simulink model "Sim_quadrotor"  (R2024a)
settings: Solver=ode4  StartTime=0.0  StopTime=18  FixedStep=sample_time_continous  RelTol=1e-3
values from neighbouring files (symbols this model uses):
  A_continuous = [0,0,0,1,0,0,0,0,0,0,0,0;      0,0,0,0,1,0,0,0,0,0,0,0;      0,0,0,0,0,1,0,0,0,0,0,0;      0,0,0,0,0,0,g * sin(alpha),g * cos(alpha),0,0,0,0;      0,0,0,0,0,0,-g * cos(alpha),g * sin(alpha),0,0,0,0;      0,0,0,0,0,0,0,0,0,0,0,0;      0,0,0,0,0,0,0,0,0,1,0,0;      0,0,0,0,0,0,0,0,0,0,1,0;      0,0,0,0,0,0,0,0,0,0,0,1;      0,0,0,0,0,0,0,0,0,0,0,0;      0,0,0,0,0,0,0,0,0,0,0,0;      0,0,0,0,0,0,0,0, ...(+8 chars)    [Main_quadrotor.m]
  A_continuous_outer = [zeros(3, 3), eye(3)     , zeros(3, 3);                       zeros(3, 3), zeros(3, 3), G          ;                       zeros(3, 3), zeros(3, 3), zeros(3, 3)]    [Main_quadrotor.m]
  B_continuous = [0,0,0,0;      0,0,0,0;      0,0,0,0;      0,0,0,0;      0,0,0,0;      1/m,1/m,1/m,1/m;      0,0,0,0;      0,0,0,0;      0,0,0,0;      inertia_true_inverse*[layout_true(2,:);-layout_true(1,:);layout_true(3,:)]]    [Main_quadrotor.m]
  B_continuous_outer = [zeros(5, 1), zeros(5, 3);                       1/m        , zeros(1, 3);                       zeros(3, 1), eye(3)     ]    [Main_quadrotor.m]
  C_inner_and_outer = eye(12)    [Main_quadrotor.m]
  DSM_val_lower_threshold_pathFG = 0    [Main_quadrotor.m]
  DSM_val_upper_threshold_pathFG = 0.01    [Main_quadrotor.m]
  goal = [2.5; 2.5; 1]    [Main_quadrotor.m]
  inner_controller_inclusion = 0    [Main_quadrotor.m]
  iter_max_pathFG = 50    [Main_quadrotor.m]
  K_lqr_outer_loop = K_lqr_outer_loop_discrete_time    [Main_quadrotor.m]
  kappa_o = 5    [Main_quadrotor.m]
  kappa_pathFG = 0.5    [Main_quadrotor.m]
  kappa_s = 2    [Main_quadrotor.m]
  MPC_max_iters = 200    [Main_quadrotor.m]
  nrotor_initial_condition = [start; zeros(9, 1)]    [Main_quadrotor.m]
  obstacle_sizes = obstacle_sizes'    [Main_quadrotor.m]
  obstacles = obstacles'    [Main_quadrotor.m]
  PathFG_max_N = 30    [Main_quadrotor.m]
  prediction_horizon_MPC = prediction_horizons_MPC(1)    [Main_quadrotor.m]
  safety_margin_universal = 0.05    [Main_quadrotor.m]
  sample_time_controller_outer = 1/10    (= 0.1)    [Main_quadrotor.m]    (also in Main_unicycle.m)
  sample_time_pathFG = sample_time_controller_outer    (= 0.1)    [Main_quadrotor.m]    (also in Main_unicycle.m)
  solver = 2    [Main_quadrotor.m]
  start = [0.1; 0.1; 0.3]    [Main_quadrotor.m]
  u_max = [thrust_max - mass_true * g; 0.5*pi; 0.5*pi; 0.5*pi]    [Main_quadrotor.m]
  u_min = [thrust_min - mass_true * g + thrust_space_saved_for_PID_inner_controller; -0.5*pi; -0.5*pi; -0.5*pi]    [Main_quadrotor.m]
undefined symbols (not defined in the file or in its folder): agent_params, agent_size, cmd_2_newtons_conversion_linear_coefficient, cmd_2_newtons_conversion_quadratic_coefficient, cmd_max, cmd_min, constr_mat, decision_variables_init, DiscIntNeverNeededParam, g, inertia_true, inertia_true_inverse, K_lqr_outer_loop_discrete_time, layout_true, mass_for_controller, mass_true, measurement_noise_accelerometer_covariance_decomposition, measurement_noise_accelerometer_mean, measurement_noise_accelerometer_seed, measurement_noise_accelerometer_var, measurement_noise_body_accelerations_inclusion_multiplier, measurement_noise_body_rates_inclusion_multiplier, measurement_noise_full_state_inclusion_multiplier, measurement_noise_full_state_mean, measurement_noise_full_state_seed, measurement_noise_full_state_var, measurement_noise_gyroscope_covariance_decomposition, measurement_noise_gyroscope_mean, measurement_noise_gyroscope_seed, measurement_noise_gyroscope_var, nrotor_vehicle_thrust_max, obs_params, P_matrix, path, pid_x_body_rate_integrator_limit, pid_x_body_rate_kp, pid_y_body_rate_integrator_limit, pid_y_body_rate_kp, pid_z_body_rate_kp, rect_obs, sample_time_controller_inner, sample_time_measurements_body_accelerations, sample_time_measurements_body_rates, sample_time_measurements_full_state, size_of_path, ssmodel, weights
libraries: simulink x15
settings Model: Creator=NewCrest Consulting  LastModifiedBy=serena
settings RTWCC: GPUComputeCapability=3.5

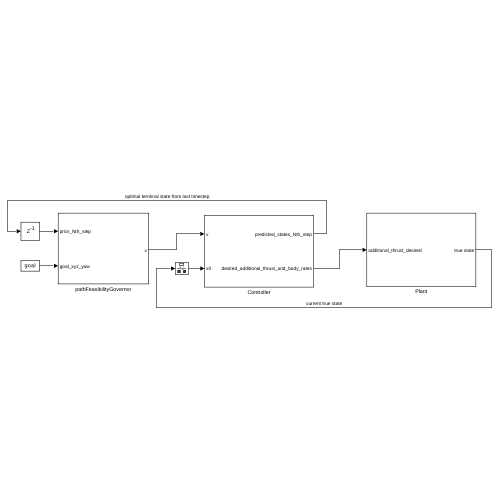
[thumbnail: Simulink's stored preview of the top-level diagram]
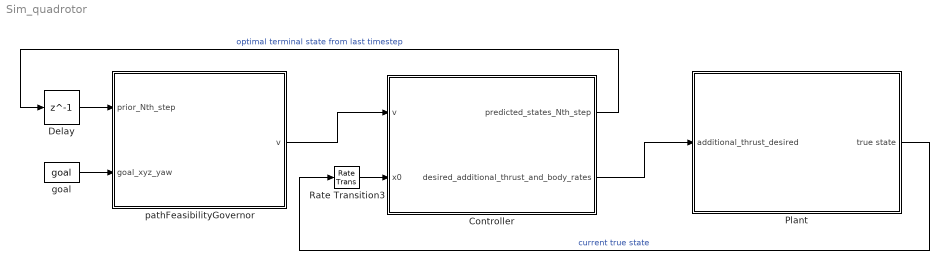
== system Sim_quadrotor ==
  Controller : Subsystem
  Delay : Delay  DelayLength=1  InitialCondition=[start;0;0;0;0;0;0]
  Plant : Subsystem
  Rate Transition3 : RateTransition  InitialCondition=[start;0;0;0;0;0;0]  OutPortSampleTime=sample_time_controller_outer
  goal : Constant  Value=goal
  pathFeasibilityGovernor : Subsystem  VariantControl=ref_source == 3
  wires:
  goal/1 -> pathFeasibilityGovernor/2(goal_xyz_yaw)
  Rate Transition3/1 -> Controller/2(x0)
  Plant/1(true state) -> Rate Transition3/1  "current true state"
  Delay/1 -> pathFeasibilityGovernor/1(prior_Nth_step)
  pathFeasibilityGovernor/1(v) -> Controller/1(v)
  Controller/1(predicted_states_Nth_step) -> Delay/1  "optimal terminal state from last timestep"
  Controller/2(desired_additional_thrust_and_body_rates) -> Plant/1(additional_thrust_desired)

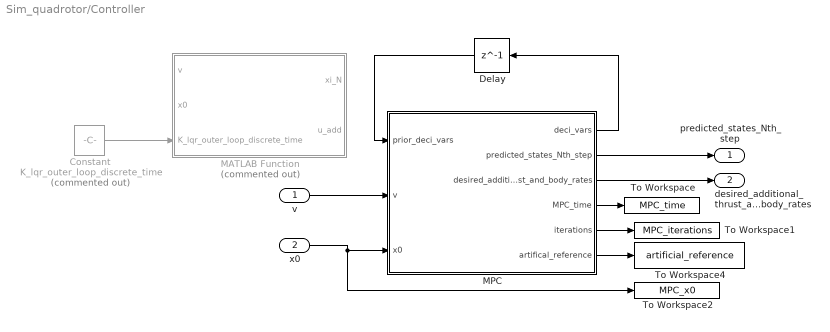
== system Sim_quadrotor/Controller ==
  v : Inport
  x0 : Inport  Port=2
  Constant : Constant  Commented=on  Value=K_lqr_outer_loop_discrete_time
  Delay : Delay  DelayLength=1  InitialCondition=decision_variables_init
  MATLAB Function : MATLAB Function  Commented=on  TreatAsAtomicUnit=on
  MPC : MATLAB Function  TreatAsAtomicUnit=on  SystemSampleTime=sample_time_controller_outer
  To Workspace : ToWorkspace  VariableName=MPC_time  SaveFormat=Timeseries  SampleTime=-1
  To Workspace1 : ToWorkspace  VariableName=MPC_iterations  SaveFormat=Timeseries  SampleTime=-1
  To Workspace2 : ToWorkspace  VariableName=MPC_x0  SaveFormat=Timeseries  SampleTime=-1
  To Workspace4 : ToWorkspace  VariableName=artificial_reference  SaveFormat=Timeseries  SampleTime=-1
  predicted_states_Nth_step : Outport
  desired_additional_thrust_and_body_rates : Outport  Port=2
  wires:
  Delay/1 -> MPC/1(prior_deci_vars)
  MPC/1(deci_vars) -> Delay/1
  v/1 -> MPC/2(v)
  MPC/2(predicted_states_Nth_step) -> predicted_states_Nth_step/1
  x0/1 -> To Workspace2/1, MPC/3(x0)
  MPC/3(desired_additional_thrust_and_body_rates) -> desired_additional_thrust_and_body_rates/1
  Constant/1 -> MATLAB Function/3(K_lqr_outer_loop_discrete_time)
  MPC/4(MPC_time) -> To Workspace/1
  MPC/5(iterations) -> To Workspace1/1
  MPC/6(artifical_reference) -> To Workspace4/1

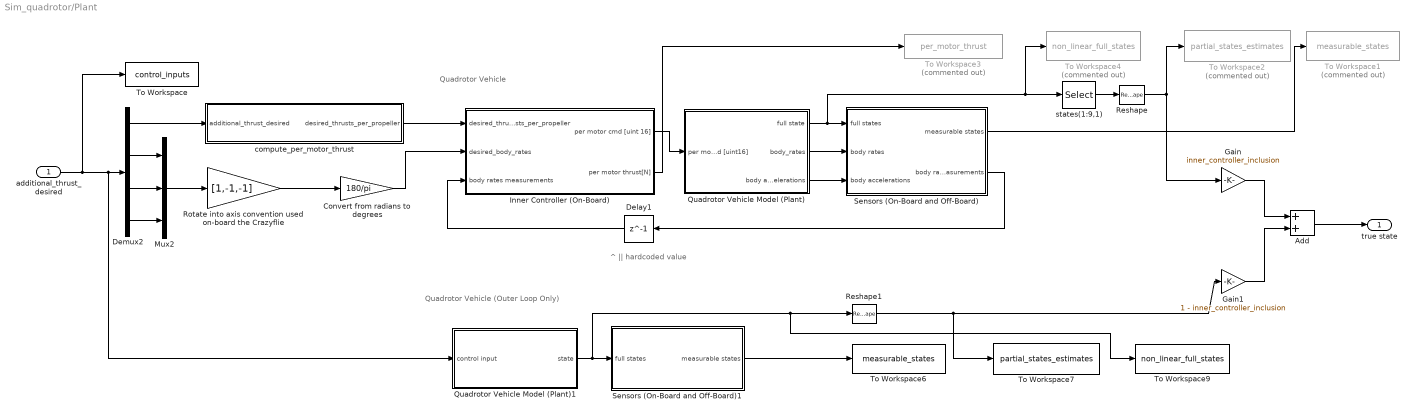
== system Sim_quadrotor/Plant ==
  note: Quadrotor Vehicle
  note: ^
      |             ||
      | hardcoded value
  note: Quadrotor Vehicle (Outer Loop Only)
  additional_thrust_desired : Inport
  Add : Sum
  Convert from radians to degrees : Gain  Gain=180/pi
  Delay1 : Delay  DelayLength=1  InitialCondition=[0;0;0]
  Demux2 : Demux
  Gain : Gain  Gain=inner_controller_inclusion
  Gain1 : Gain  Gain=1 - inner_controller_inclusion
  Inner Controller (On-Board) : Subsystem
  Mux2 : Mux  Inputs=3
  Quadrotor Vehicle Model (Plant) : Subsystem
  Quadrotor Vehicle Model (Plant)1 : Subsystem
  Reshape : Reshape  OutputDimensionality=Column vector (2-D)
  Reshape1 : Reshape  OutputDimensionality=Column vector (2-D)
  Rotate into axis convention used on-board the Crazyflie : Gain  Gain=[1,-1,-1]
  Sensors (On-Board and Off-Board) : Subsystem
  Sensors (On-Board and Off-Board)1 : Subsystem
  To Workspace : ToWorkspace  VariableName=control_inputs  SaveFormat=Timeseries  SampleTime=-1
  To Workspace1 : ToWorkspace  Commented=on  VariableName=measurable_states  SaveFormat=Timeseries  SampleTime=-1
  To Workspace2 : ToWorkspace  Commented=on  VariableName=partial_states_estimates  SaveFormat=Timeseries  SampleTime=-1
  To Workspace3 : ToWorkspace  Commented=on  VariableName=per_motor_thrust  SaveFormat=Timeseries  SampleTime=-1
  To Workspace4 : ToWorkspace  Commented=on  VariableName=non_linear_full_states  SaveFormat=Timeseries  SampleTime=-1
  To Workspace6 : ToWorkspace  VariableName=measurable_states  SaveFormat=Timeseries  SampleTime=-1
  To Workspace7 : ToWorkspace  VariableName=partial_states_estimates  SaveFormat=Timeseries  SampleTime=-1
  To Workspace9 : ToWorkspace  VariableName=non_linear_full_states  SaveFormat=Timeseries  SampleTime=-1
  compute_per_motor_thrust : MATLAB Function  TreatAsAtomicUnit=on
  states(1:9,1) : Selector  InputPortWidth=12  IndexOptions=Index vector (dialog)  Indices=[1,2,3,4,5,6,7,8,9]  OutputSizes=1
  true state : Outport
  wires:
  Sensors (On-Board and Off-Board)/1(measurable states) -> To Workspace1/1
  Quadrotor Vehicle Model (Plant)/3(body accelerations) -> Sensors (On-Board and Off-Board)/3(body accelerations)
  Inner Controller (On-Board)/2(per motor thrust[N]) -> To Workspace3/1
  Quadrotor Vehicle Model (Plant)/2(body_rates) -> Sensors (On-Board and Off-Board)/2(body rates)
  Inner Controller (On-Board)/1(per motor cmd [uint 16]) -> Quadrotor Vehicle Model (Plant)/1(per motor cmd [uint16])
  compute_per_motor_thrust/1(desired_thrusts_per_propeller) -> Inner Controller (On-Board)/1(desired_thrusts_per_propeller)
  Convert from radians to degrees/1 -> Inner Controller (On-Board)/2(desired_body_rates)
  Rotate into axis convention used on-board the Crazyflie/1 -> Convert from radians to degrees/1
  additional_thrust_desired/1 -> Quadrotor Vehicle Model (Plant)1/1(control input), Demux2/1, To Workspace/1
  Demux2/1 -> compute_per_motor_thrust/1(additional_thrust_desired)
  Demux2/2 -> Mux2/1
  Demux2/4 -> Mux2/3
  Demux2/3 -> Mux2/2
  Mux2/1 -> Rotate into axis convention used on-board the Crazyflie/1
  Quadrotor Vehicle Model (Plant)/1(full state) -> Sensors (On-Board and Off-Board)/1(full states), To Workspace4/1, states(1:9,1)/1
  Reshape/1 -> Gain/1, To Workspace2/1
  states(1:9,1)/1 -> Reshape/1
  Sensors (On-Board and Off-Board)/2(body rates measurements) -> Delay1/1
  Delay1/1 -> Inner Controller (On-Board)/3(body rates measurements)
  Sensors (On-Board and Off-Board)1/1(measurable states) -> To Workspace6/1
  Reshape1/1 -> Gain1/1, To Workspace7/1
  Quadrotor Vehicle Model (Plant)1/1(state) -> Sensors (On-Board and Off-Board)1/1(full states), Reshape1/1, To Workspace9/1
  Gain/1 -> Add/1
  Gain1/1 -> Add/2
  Add/1 -> true state/1

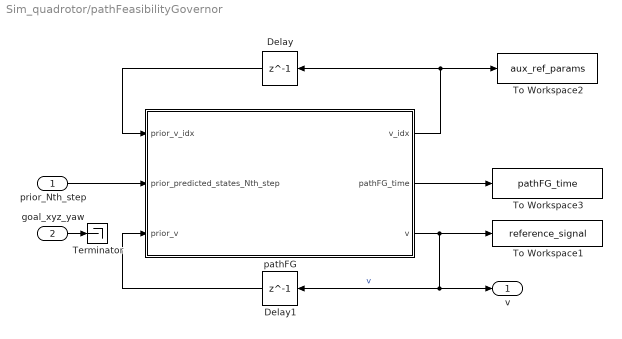
== system Sim_quadrotor/pathFeasibilityGovernor ==
  prior_Nth_step : Inport
  goal_xyz_yaw : Inport  Port=2
  Delay : Delay  DelayLength=1  InitialCondition=1
  Delay1 : Delay  DelayLength=1  InitialCondition=[start;0]
  Terminator : Terminator
  To Workspace1 : ToWorkspace  VariableName=reference_signal  SaveFormat=Timeseries  SampleTime=-1
  To Workspace2 : ToWorkspace  VariableName=aux_ref_params  SaveFormat=Timeseries  SampleTime=-1
  To Workspace3 : ToWorkspace  VariableName=pathFG_time  SaveFormat=Timeseries  SampleTime=-1
  pathFG : MATLAB Function  TreatAsAtomicUnit=on  SystemSampleTime=sample_time_pathFG
  v : Outport
  wires:
  goal_xyz_yaw/1 -> Terminator/1
  pathFG/3(v) -> To Workspace1/1, v/1, Delay1/1  "v"
  prior_Nth_step/1 -> pathFG/2(prior_predicted_states_Nth_step)
  pathFG/1(v_idx) -> Delay/1, To Workspace2/1
  Delay/1 -> pathFG/1(prior_v_idx)
  Delay1/1 -> pathFG/3(prior_v)
  pathFG/2(pathFG_time) -> To Workspace3/1

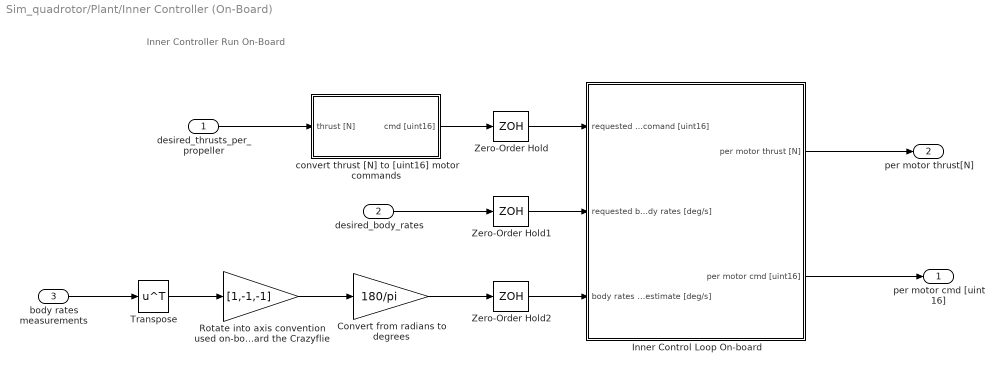
== system Sim_quadrotor/Plant/Inner Controller (On-Board) ==
  note: Inner Controller Run On-Board
  desired_thrusts_per_propeller : Inport
  desired_body_rates : Inport  Port=2
  body rates measurements : Inport  Port=3
  Convert from radians to degrees : Gain  Gain=180/pi
  Inner Control Loop On-board : Subsystem
  Rotate into axis convention used on-board the Crazyflie : Gain  Gain=[1,-1,-1]
  Transpose : Math  Operator=transpose
  Zero-Order Hold : ZeroOrderHold  SampleTime=sample_time_controller_inner
  Zero-Order Hold1 : ZeroOrderHold  SampleTime=sample_time_controller_inner
  Zero-Order Hold2 : ZeroOrderHold  SampleTime=sample_time_controller_inner
  convert thrust [N] to [uint16] motor commands : Subsystem
  per motor cmd [uint 16] : Outport
  per motor thrust[N] : Outport  Port=2
  wires:
  Inner Control Loop On-board/2(per motor cmd [uint16]) -> per motor cmd [uint 16]/1
  desired_body_rates/1 -> Zero-Order Hold1/1
  Zero-Order Hold/1 -> Inner Control Loop On-board/1(requested per motor comand [uint16])
  desired_thrusts_per_propeller/1 -> convert thrust [N] to [uint16] motor commands/1(thrust [N])
  Zero-Order Hold2/1 -> Inner Control Loop On-board/3(body rates estimate [deg/s])
  Zero-Order Hold1/1 -> Inner Control Loop On-board/2(requested body rates [deg/s])
  Inner Control Loop On-board/1(per motor thrust [N]) -> per motor thrust[N]/1
  Rotate into axis convention used on-board the Crazyflie/1 -> Convert from radians to degrees/1
  Convert from radians to degrees/1 -> Zero-Order Hold2/1
  body rates measurements/1 -> Transpose/1
  convert thrust [N] to [uint16] motor commands/1(cmd [uint16]) -> Zero-Order Hold/1
  Transpose/1 -> Rotate into axis convention used on-board the Crazyflie/1

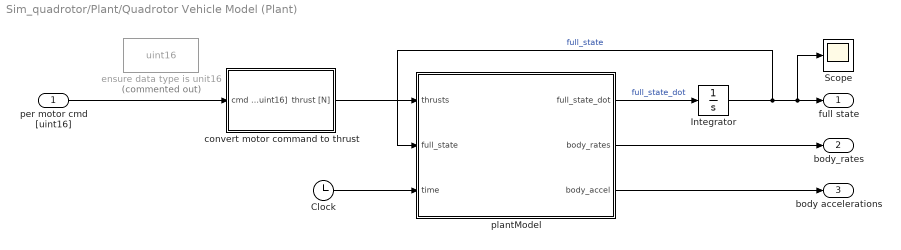
== system Sim_quadrotor/Plant/Quadrotor Vehicle Model (Plant) ==
  per motor cmd [uint16] : Inport
  Clock : Clock
  Integrator : Integrator  InitialCondition=nrotor_initial_condition
  Scope : Scope
  convert motor command to thrust : Subsystem
  ensure data type is unit16 : DataTypeConversion  Commented=on  OutDataTypeStr=uint16  SaturateOnIntegerOverflow=off  RndMeth=Floor
  plantModel : MATLAB Function  TreatAsAtomicUnit=on
  full state : Outport  VectorParamsAs1DForOutWhenUnconnected=off
  body_rates : Outport  Port=2  VectorParamsAs1DForOutWhenUnconnected=off
  body accelerations : Outport  Port=3  VectorParamsAs1DForOutWhenUnconnected=off
  wires:
  plantModel/3(body_accel) -> body accelerations/1
  convert motor command to thrust/1(thrust [N]) -> plantModel/1(thrusts)
  plantModel/2(body_rates) -> body_rates/1
  plantModel/1(full_state_dot) -> Integrator/1  "full_state_dot"
  per motor cmd [uint16]/1 -> convert motor command to thrust/1(cmd [uint16])
  Integrator/1 -> Scope/1, full state/1, plantModel/2(full_state)  "full_state"
  Clock/1 -> plantModel/3(time)

== system Sim_quadrotor/Plant/Quadrotor Vehicle Model (Plant)1 ==
  control input : Inport
  Integrator : Integrator  InitialCondition=nrotor_initial_condition(1:9)
  MATLAB Function : MATLAB Function  TreatAsAtomicUnit=on
  Scope : Scope
  state : Outport  VectorParamsAs1DForOutWhenUnconnected=off
  wires:
  control input/1 -> MATLAB Function/2(control_input)
  MATLAB Function/1(state_dot) -> Integrator/1  "state_dot"
  Integrator/1 -> Scope/1, MATLAB Function/1(state), state/1  "state"

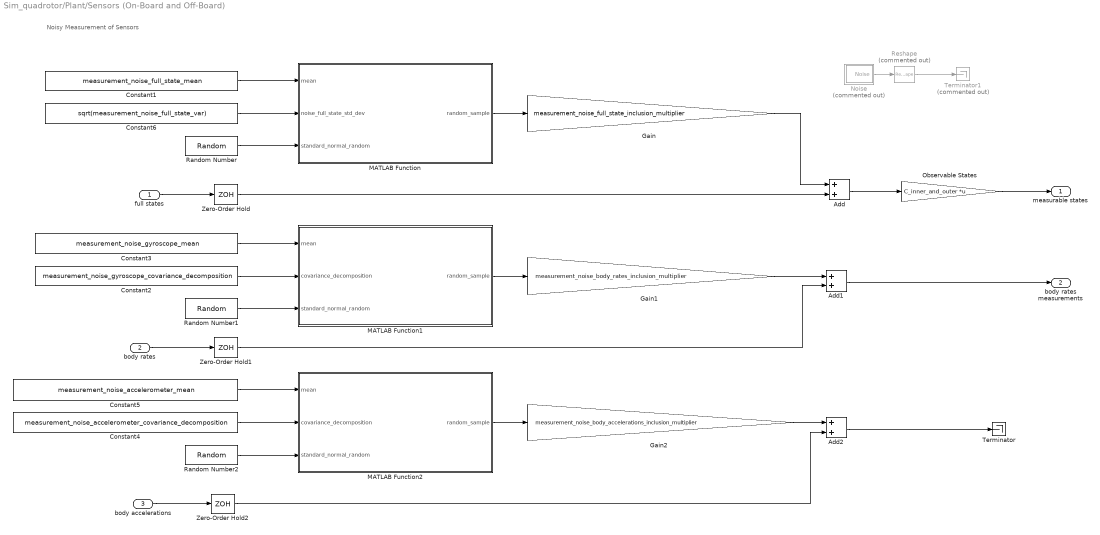
== system Sim_quadrotor/Plant/Sensors (On-Board and Off-Board) ==
  note: Noisy Measurement of Sensors
  full states : Inport
  body rates : Inport  Port=2
  body accelerations : Inport  Port=3
  Add : Sum
  Add1 : Sum
  Add2 : Sum
  Constant1 : Constant  Value=measurement_noise_full_state_mean  VectorParams1D=off
  Constant2 : Constant  Value=measurement_noise_gyroscope_covariance_decomposition
  Constant3 : Constant  Value=measurement_noise_gyroscope_mean
  Constant4 : Constant  Value=measurement_noise_accelerometer_covariance_decomposition
  Constant5 : Constant  Value=measurement_noise_accelerometer_mean
  Constant6 : Constant  Value=sqrt(measurement_noise_full_state_var)
  Gain : Gain  Gain=measurement_noise_full_state_inclusion_multiplier
  Gain1 : Gain  Gain=measurement_noise_body_rates_inclusion_multiplier
  Gain2 : Gain  Gain=measurement_noise_body_accelerations_inclusion_multiplier
  MATLAB Function : MATLAB Function  TreatAsAtomicUnit=on
  MATLAB Function1 : MATLAB Function  TreatAsAtomicUnit=on
  MATLAB Function2 : MATLAB Function  TreatAsAtomicUnit=on
  Noise : Subsystem  Commented=on
  Observable States : Gain  Gain=C_inner_and_outer  Multiplication=Matrix(K*u)
  Random Number : RandomNumber  Mean=zeros(12,1)  Variance=ones(12,1)  Seed=measurement_noise_full_state_seed  SampleTime=sample_time_measurements_full_state  VectorParams1D=off
  Random Number1 : RandomNumber  Mean=measurement_noise_gyroscope_mean  Variance=measurement_noise_gyroscope_var  Seed=measurement_noise_gyroscope_seed  SampleTime=sample_time_measurements_body_rates  VectorParams1D=off
  Random Number2 : RandomNumber  Mean=measurement_noise_accelerometer_mean  Variance=measurement_noise_accelerometer_var  Seed=measurement_noise_accelerometer_seed  SampleTime=sample_time_measurements_body_accelerations  VectorParams1D=off
  Reshape : Reshape  Commented=on  OutputDimensionality=Column vector (2-D)
  Terminator : Terminator
  Terminator1 : Terminator  Commented=on
  Zero-Order Hold : ZeroOrderHold  SampleTime=sample_time_measurements_full_state
  Zero-Order Hold1 : ZeroOrderHold  SampleTime=sample_time_measurements_body_rates
  Zero-Order Hold2 : ZeroOrderHold  SampleTime=sample_time_measurements_body_accelerations
  measurable states : Outport
  body rates measurements : Outport  Port=2
  wires:
  full states/1 -> Zero-Order Hold/1
  body rates/1 -> Zero-Order Hold1/1
  body accelerations/1 -> Zero-Order Hold2/1
  Zero-Order Hold/1 -> Add/2
  Zero-Order Hold1/1 -> Add1/2
  Zero-Order Hold2/1 -> Add2/2
  Random Number/1 -> MATLAB Function/3(standard_normal_random)
  Constant1/1 -> MATLAB Function/1(mean)
  MATLAB Function/1(random_sample) -> Gain/1
  Gain/1 -> Add/1
  Random Number1/1 -> MATLAB Function1/3(standard_normal_random)
  Gain1/1 -> Add1/1
  Constant3/1 -> MATLAB Function1/1(mean)
  Constant2/1 -> MATLAB Function1/2(covariance_decomposition)
  MATLAB Function1/1(random_sample) -> Gain1/1
  MATLAB Function2/1(random_sample) -> Gain2/1
  Random Number2/1 -> MATLAB Function2/3(standard_normal_random)
  Gain2/1 -> Add2/1
  Constant4/1 -> MATLAB Function2/2(covariance_decomposition)
  Constant5/1 -> MATLAB Function2/1(mean)
  Add2/1 -> Terminator/1
  Add1/1 -> body rates measurements/1
  Add/1 -> Observable States/1
  Observable States/1 -> measurable states/1
  Noise/1(Noise) -> Reshape/1
  Reshape/1 -> Terminator1/1
  Constant6/1 -> MATLAB Function/2(noise_full_state_std_dev)

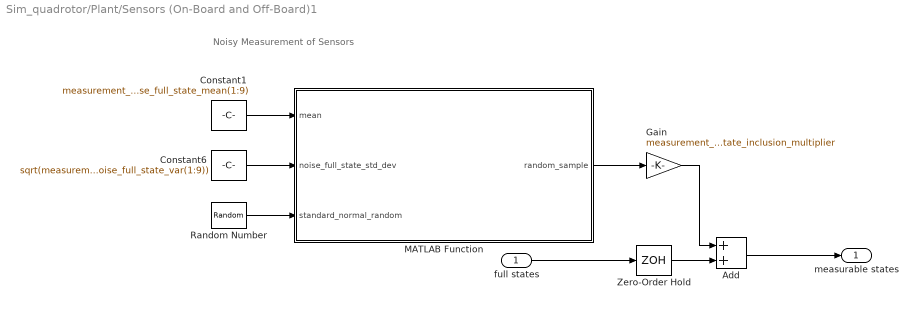
== system Sim_quadrotor/Plant/Sensors (On-Board and Off-Board)1 ==
  note: Noisy Measurement of Sensors
  full states : Inport
  Add : Sum
  Constant1 : Constant  Value=measurement_noise_full_state_mean(1:9)  VectorParams1D=off
  Constant6 : Constant  Value=sqrt(measurement_noise_full_state_var(1:9))
  Gain : Gain  Gain=measurement_noise_full_state_inclusion_multiplier
  MATLAB Function : MATLAB Function  TreatAsAtomicUnit=on
  Random Number : RandomNumber  Mean=zeros(9,1)  Variance=ones(9,1)  Seed=measurement_noise_full_state_seed(1:9)  SampleTime=sample_time_measurements_full_state  VectorParams1D=off
  Zero-Order Hold : ZeroOrderHold  SampleTime=sample_time_measurements_full_state
  measurable states : Outport
  wires:
  full states/1 -> Zero-Order Hold/1
  Zero-Order Hold/1 -> Add/2
  Constant6/1 -> MATLAB Function/2(noise_full_state_std_dev)
  Gain/1 -> Add/1
  Random Number/1 -> MATLAB Function/3(standard_normal_random)
  MATLAB Function/1(random_sample) -> Gain/1
  Constant1/1 -> MATLAB Function/1(mean)
  Add/1 -> measurable states/1

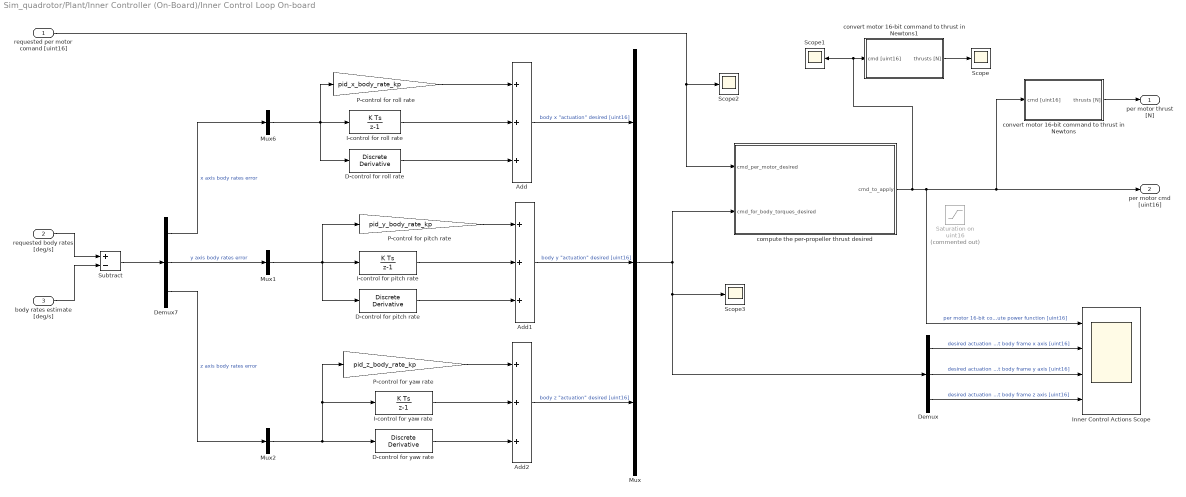
== system Sim_quadrotor/Plant/Inner Controller (On-Board)/Inner Control Loop On-board ==
  requested per motor comand [uint16] : Inport
  requested body rates [deg/s] : Inport  Port=2
  body rates estimate [deg/s] : Inport  Port=3
  Add : Sum  Inputs=+++
  Add1 : Sum  Inputs=+++
  Add2 : Sum  Inputs=+++
  D-control for pitch rate : simulink/Discrete/Discrete Derivative  gainval=pid_y_body_rate_kd  ICPrevScaledInput=0.0  OutMin=[]  OutMax=[]  OutDataType=fixdt(1, 16)  OutScaling=2^-10  DoSatur=off
  D-control for roll rate : simulink/Discrete/Discrete Derivative  gainval=pid_x_body_rate_kd  ICPrevScaledInput=0.0  OutMin=[]  OutMax=[]  OutDataType=fixdt(1, 16)  OutScaling=2^-10  DoSatur=off
  D-control for yaw rate : simulink/Discrete/Discrete Derivative  gainval=pid_z_body_rate_kd  ICPrevScaledInput=0.0  OutMin=[]  OutMax=[]  OutDataType=fixdt(1, 16)  OutScaling=2^-10  DoSatur=off
  Demux : Demux  Outputs=3
  Demux7 : Demux  Outputs=3
  I-control for pitch rate : DiscreteIntegrator  gainval=pid_y_body_rate_ki  SampleTime=-1  LimitOutput=on  UpperSaturationLimit=pid_y_body_rate_integrator_limit  LowerSaturationLimit=-pid_y_body_rate_integrator_limit  ICPrevOutput=DiscIntNeverNeededParam  ICPrevScaledInput=DiscIntNeverNeededParam
  I-control for roll rate : DiscreteIntegrator  gainval=pid_x_body_rate_ki  SampleTime=-1  LimitOutput=on  UpperSaturationLimit=pid_x_body_rate_integrator_limit  LowerSaturationLimit=-pid_x_body_rate_integrator_limit  ICPrevOutput=DiscIntNeverNeededParam  ICPrevScaledInput=DiscIntNeverNeededParam
  I-control for yaw rate : DiscreteIntegrator  gainval=pid_z_body_rate_ki  SampleTime=-1  LimitOutput=on  UpperSaturationLimit=pid_x_body_rate_integrator_limit  LowerSaturationLimit=-pid_x_body_rate_integrator_limit  ICPrevOutput=DiscIntNeverNeededParam  ICPrevScaledInput=DiscIntNeverNeededParam
  Inner Control Actions Scope : Scope  NumInputPorts=4
  Mux : Mux  Inputs=3
  Mux1 : Mux  Inputs=1
  Mux2 : Mux  Inputs=1
  Mux6 : Mux  Inputs=1
  P-control for pitch rate : Gain  Gain=pid_y_body_rate_kp
  P-control for roll rate : Gain  Gain=pid_x_body_rate_kp
  P-control for yaw rate : Gain  Gain=pid_z_body_rate_kp
  Saturation on uint16 : Saturate  Commented=on  UpperLimit=cmd_max  LowerLimit=cmd_min  ZeroCross=off
  Scope{,1..3} (4 alike) : Scope
  Subtract : Sum  Inputs=+-
  compute the per-propeller thrust desired : MATLAB Function  TreatAsAtomicUnit=on
  convert motor 16-bit command to thrust in Newtons : Subsystem
  convert motor 16-bit command to thrust in Newtons1 : Subsystem
  per motor thrust [N] : Outport  VectorParamsAs1DForOutWhenUnconnected=off
  per motor cmd [uint16] : Outport  Port=2  VectorParamsAs1DForOutWhenUnconnected=off
  wires:
  Demux/3 -> Inner Control Actions Scope/4  "desired actuation about body frame z axis [uint16]"
  P-control for pitch rate/1 -> Add1/1
  D-control for roll rate/1 -> Add/3
  Demux7/2 -> Mux1/1  "y axis body rates error"
  Mux/1 -> compute the per-propeller thrust desired/2(cmd_for_body_torques_desired), Scope3/1, Demux/1
  requested body rates [deg/s]/1 -> Subtract/1
  Mux6/1 -> D-control for roll rate/1, I-control for roll rate/1, P-control for roll rate/1
  Subtract/1 -> Demux7/1
  I-control for roll rate/1 -> Add/2
  body rates estimate [deg/s]/1 -> Subtract/2
  compute the per-propeller thrust desired/1(cmd_to_apply) -> Scope1/1, convert motor 16-bit command to thrust in Newtons1/1(cmd [uint16]), per motor cmd [uint16]/1, convert motor 16-bit command to thrust in Newtons/1(cmd [uint16]), Inner Control Actions Scope/1  "per motor 16-bit command after distribute power function [uint16]"
  requested per motor comand [uint16]/1 -> compute the per-propeller thrust desired/1(cmd_per_motor_desired), Scope2/1
  convert motor 16-bit command to thrust in Newtons/1(thrusts [N]) -> per motor thrust [N]/1
  Add1/1 -> Mux/2  "body y \"actuation\" desired [uint16]"
  Demux7/1 -> Mux6/1  "x axis body rates error"
  I-control for pitch rate/1 -> Add1/2
  Demux/1 -> Inner Control Actions Scope/2  "desired actuation about body frame x axis [uint16]"
  Add2/1 -> Mux/3  "body z \"actuation\" desired [uint16]"
  Mux1/1 -> D-control for pitch rate/1, P-control for pitch rate/1, I-control for pitch rate/1
  Mux2/1 -> I-control for yaw rate/1, P-control for yaw rate/1, D-control for yaw rate/1
  Demux7/3 -> Mux2/1  "z axis body rates error"
  Add/1 -> Mux/1  "body x \"actuation\" desired [uint16]"
  P-control for roll rate/1 -> Add/1
  D-control for yaw rate/1 -> Add2/3
  I-control for yaw rate/1 -> Add2/2
  D-control for pitch rate/1 -> Add1/3
  P-control for yaw rate/1 -> Add2/1
  Demux/2 -> Inner Control Actions Scope/3  "desired actuation about body frame y axis [uint16]"
  convert motor 16-bit command to thrust in Newtons1/1(thrusts [N]) -> Scope/1

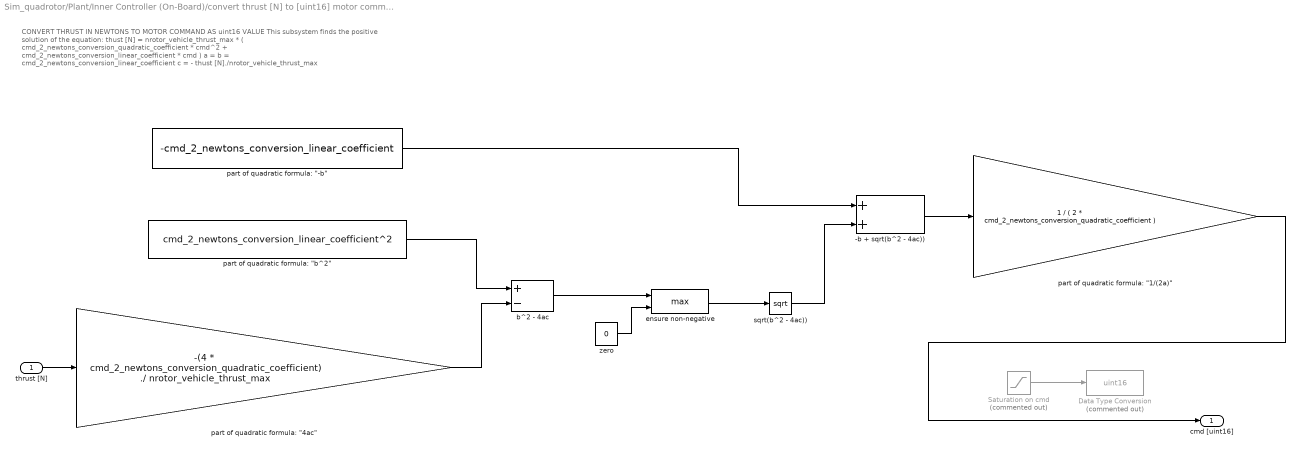
== system Sim_quadrotor/Plant/Inner Controller (On-Board)/convert thrust [N] to [uint16] motor commands ==
  note: CONVERT THRUST IN NEWTONS TO MOTOR COMMAND AS uint16 VALUE
      | This subsystem finds the positive solution of the equation:
      | thust [N] = nrotor_vehicle_thrust_max * ( cmd_2_newtons_conversion_quadratic_coefficient * cmd^2 + cmd_2_newtons_conversion_linear_coefficient * cmd )
      | a = b = cmd_2_newtons_conversion_linear_coefficient
      | c = - thust [N]./nrotor_vehicle_thrust_max
  thrust [N] : Inport
  -b + sqrt(b^2 - 4ac)) : Sum
  Data Type Conversion : DataTypeConversion  Commented=on  OutDataTypeStr=uint16  SaturateOnIntegerOverflow=off  RndMeth=Floor
  Saturation on cmd : Saturate  Commented=on  UpperLimit=cmd_max  LowerLimit=cmd_min  ZeroCross=off
  b^2 - 4ac : Sum  Inputs=+-
  ensure non-negative : MinMax  Function=max  Inputs=2
  "part of quadratic formula: \"-b\"" : Constant  Value=-cmd_2_newtons_conversion_linear_coefficient
  "part of quadratic formula: \"1/(2a)\"" : Gain  Gain=1 / ( 2 * cmd_2_newtons_conversion_quadratic_coefficient )
  "part of quadratic formula: \"4ac\"" : Gain  Gain=-(4 * cmd_2_newtons_conversion_quadratic_coefficient) ./ nrotor_vehicle_thrust_max
  "part of quadratic formula: \"b^2\"" : Constant  Value=cmd_2_newtons_conversion_linear_coefficient^2
  sqrt(b^2 - 4ac)) : Sqrt
  zero : Constant  Value=0
  cmd [uint16] : Outport  VectorParamsAs1DForOutWhenUnconnected=off
  wires:
  thrust [N]/1 -> "part of quadratic formula: \"4ac\""/1
  Saturation on cmd/1 -> Data Type Conversion/1
  "part of quadratic formula: \"4ac\""/1 -> b^2 - 4ac/2
  "part of quadratic formula: \"b^2\""/1 -> b^2 - 4ac/1
  b^2 - 4ac/1 -> ensure non-negative/1
  ensure non-negative/1 -> sqrt(b^2 - 4ac))/1
  "part of quadratic formula: \"-b\""/1 -> -b + sqrt(b^2 - 4ac))/1
  sqrt(b^2 - 4ac))/1 -> -b + sqrt(b^2 - 4ac))/2
  -b + sqrt(b^2 - 4ac))/1 -> "part of quadratic formula: \"1/(2a)\""/1
  "part of quadratic formula: \"1/(2a)\""/1 -> cmd [uint16]/1
  zero/1 -> ensure non-negative/2

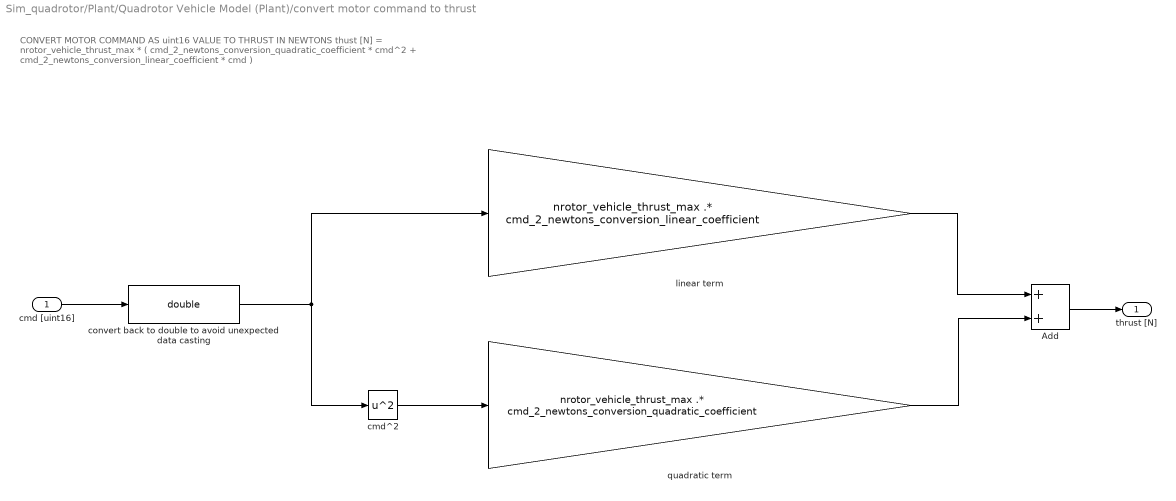
== system Sim_quadrotor/Plant/Quadrotor Vehicle Model (Plant)/convert motor command to thrust ==
  note: CONVERT MOTOR COMMAND AS uint16 VALUE TO THRUST IN NEWTONS
      | thust [N] = nrotor_vehicle_thrust_max * ( cmd_2_newtons_conversion_quadratic_coefficient * cmd^2 + cmd_2_newtons_conversion_linear_coefficient * cmd )
  cmd [uint16] : Inport
  Add : Sum
  cmd^2 : Math  Operator=square  SignedPower=on
  convert back to double to avoid unexpected data casting : DataTypeConversion  OutDataTypeStr=double  SaturateOnIntegerOverflow=off  RndMeth=Floor
  linear term : Gain  Gain=nrotor_vehicle_thrust_max .* cmd_2_newtons_conversion_linear_coefficient
  quadratic term : Gain  Gain=nrotor_vehicle_thrust_max .* cmd_2_newtons_conversion_quadratic_coefficient
  thrust [N] : Outport  VectorParamsAs1DForOutWhenUnconnected=off
  wires:
  cmd^2/1 -> quadratic term/1
  quadratic term/1 -> Add/2
  linear term/1 -> Add/1
  cmd [uint16]/1 -> convert back to double to avoid unexpected data casting/1
  Add/1 -> thrust [N]/1
  convert back to double to avoid unexpected data casting/1 -> linear term/1, cmd^2/1

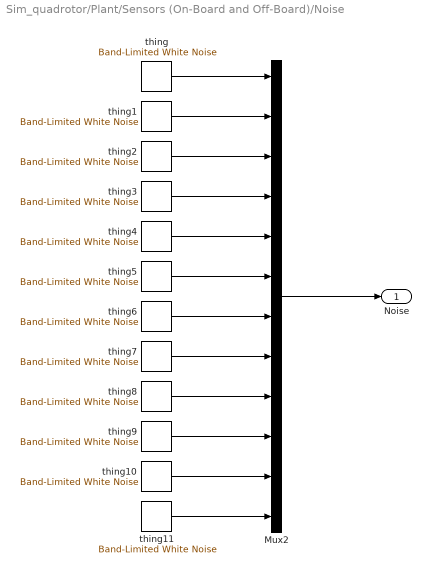
== system Sim_quadrotor/Plant/Sensors (On-Board and Off-Board)/Noise ==
  Mux2 : Mux  Inputs=12
  thing{,1..11} (12 alike) : simulink/Sources/Band-Limited White Noise  Cov=temp_noise_cov  Ts=sample_time_measurements_full_state  seed=[23341]
  Noise : Outport
  wires:
  Mux2/1 -> Noise/1
  thing/1 -> Mux2/1
  thing1/1 -> Mux2/2
  thing2/1 -> Mux2/3
  thing3/1 -> Mux2/4
  thing4/1 -> Mux2/5
  thing10/1 -> Mux2/11
  thing11/1 -> Mux2/12
  thing9/1 -> Mux2/10
  thing8/1 -> Mux2/9
  thing7/1 -> Mux2/8
  thing6/1 -> Mux2/7
  thing5/1 -> Mux2/6

== system Sim_quadrotor/Plant/Inner Controller (On-Board)/Inner Control Loop On-board/convert motor 16-bit command to thrust in Newtons ==
  note: CONVERT MOTOR COMMAND AS uint16 VALUE TO THRUST IN NEWTONS
      | Apply the following equation:
      | thust [N] = nrotor_vehicle_thrust_max * ( cmd_2_newtons_conversion_quadratic_coefficient * cmd^2 + cmd_2_newtons_conversion_linear_coefficient * cmd )
  cmd [uint16] : Inport
  Add : Sum
  cmd^2 : Math  Operator=square  SignedPower=on
  convert back to double to avoid unexpected data casting : DataTypeConversion  OutDataTypeStr=double  SaturateOnIntegerOverflow=off  RndMeth=Floor
  linear term : Gain  Gain=nrotor_vehicle_thrust_max .* cmd_2_newtons_conversion_linear_coefficient
  quadratic term : Gain  Gain=nrotor_vehicle_thrust_max .* cmd_2_newtons_conversion_quadratic_coefficient
  thrusts [N] : Outport  VectorParamsAs1DForOutWhenUnconnected=off
  wires:
  cmd^2/1 -> quadratic term/1
  quadratic term/1 -> Add/2
  linear term/1 -> Add/1
  cmd [uint16]/1 -> convert back to double to avoid unexpected data casting/1
  Add/1 -> thrusts [N]/1
  convert back to double to avoid unexpected data casting/1 -> linear term/1, cmd^2/1

== system Sim_quadrotor/Plant/Inner Controller (On-Board)/Inner Control Loop On-board/convert motor 16-bit command to thrust in Newtons1 ==
  note: CONVERT MOTOR COMMAND AS uint16 VALUE TO THRUST IN NEWTONS
      | Apply the following equation:
      | thust [N] = nrotor_vehicle_thrust_max * ( cmd_2_newtons_conversion_quadratic_coefficient * cmd^2 + cmd_2_newtons_conversion_linear_coefficient * cmd )
  cmd [uint16] : Inport
  Add : Sum
  cmd^2 : Math  Operator=square  SignedPower=on
  convert back to double to avoid unexpected data casting : DataTypeConversion  OutDataTypeStr=double  SaturateOnIntegerOverflow=off  RndMeth=Floor
  linear term : Gain  Gain=nrotor_vehicle_thrust_max .* cmd_2_newtons_conversion_linear_coefficient
  quadratic term : Gain  Gain=nrotor_vehicle_thrust_max .* cmd_2_newtons_conversion_quadratic_coefficient
  thrusts [N] : Outport  VectorParamsAs1DForOutWhenUnconnected=off
  wires:
  cmd^2/1 -> quadratic term/1
  quadratic term/1 -> Add/2
  linear term/1 -> Add/1
  cmd [uint16]/1 -> convert back to double to avoid unexpected data casting/1
  Add/1 -> thrusts [N]/1
  convert back to double to avoid unexpected data casting/1 -> linear term/1, cmd^2/1

== matlab function Sim_quadrotor/pathFeasibilityGovernor/pathFG ==
  settings: sampleTime=0.001
  data: v_idx output; pathFG_time output; mass_for_controller parameter; g parameter; u_max parameter; u_min parameter; kappa_s parameter; kappa_o parameter; obstacles parameter; obstacle_sizes parameter; agent_size parameter; K_lqr_outer_loop parameter; P_matrix parameter; kappa_pathFG parameter; iter_max_pathFG parameter; DSM_val_lower_threshold_pathFG parameter; DSM_val_upper_threshold_pathFG parameter; path parameter; prior_v_idx input; prior_predicted_states_Nth_step input; prior_v input; v output; size_of_path parameter; prediction_horizon_MPC parameter; PathFG_max_N parameter; rect_obs parameter
function [v_idx, pathFG_time, v] = callPathFG(...    
    mass_for_controller, ...
    g, ...
    u_max, ...
    u_min, ...
    kappa_s, ...
    kappa_o, ...
    obstacles, ...
    obstacle_sizes, ...
    agent_size, ...
    K_lqr_outer_loop,...
    P_matrix, ...
    kappa_pathFG, ...
    iter_max_pathFG, ...
    DSM_val_lower_threshold_pathFG, ...
    DSM_val_upper_threshold_pathFG, ...
    path, ...
    prior_v_idx, ...
    prior_predicted_states_Nth_step, ...
    prior_v, ...
    size_of_path, ...
    prediction_horizon_MPC, ...
    PathFG_max_N, rect_obs)...
    
    coder.extrinsic("pathFG");
    v_idx = 0;
    v = zeros(4, 1);

    % timer
    pathFG_start = tic;

    if (prediction_horizon_MPC >= PathFG_max_N)
        v = [reshape(path(end, :), [], 1); 0.0];
        v_idx = size_of_path;
        % disp("v");
        % disp(v);
    else
        [v_idx, v] = pathFG( ...    
            mass_for_controller, ...
            g, ...
            u_max, ...
            u_min, ...
            kappa_s, ...
            kappa_o, ...
            obstacles, ...
            obstacle_sizes, ...
            rect_obs,...
            agent_size, ...
            K_lqr_outer_loop,...
            P_matrix, ...
            kappa_pathFG, ...
            iter_max_pathFG, ...
            DSM_val_lower_threshold_pathFG, ...
            DSM_val_upper_threshold_pathFG, ...
            path, ...
            size_of_path, ...
            prior_v_idx, ...
            prior_predicted_states_Nth_step, ...
            prior_v ...
        );
    end

    pathFG_time = toc(pathFG_start);

end

== matlab function Sim_quadrotor/Controller/MPC ==
  data: prior_deci_vars input; deci_vars output; v input; x0 input; predicted_states_Nth_step output; desired_additional_thrust_and_body_rates output; ssmodel parameter; weights parameter; constr_mat parameter; solver parameter; obs_params parameter; agent_params parameter; MPC_time output; iterations output; safety_margin_universal parameter; MPC_max_iters parameter; artifical_reference output

function [deci_vars,...
          predicted_states_Nth_step,...
          desired_additional_thrust_and_body_rates,...
          MPC_time, ...
          iterations, artifical_reference] ...
          = callMPC(...
              prior_deci_vars,...
              v,...
              x0,...
              ssmodel,...
              weights,...
              constr_mat,...
              solver,...
              obs_params,...
              agent_params,...
              safety_margin_universal, ...
              MPC_max_iters)
    

    % % Note!!! In Simulink's MPC function, when solver = 3 or 5, the solve value has to be set
    % % manually because they have different decision variable dimensions compared to other
    % % solvers. Matlab check the dimension integrety using defaul solver which might
    % % cause discrepency.
    if(solver ~= 5)
    else
        solver = 5;
    end

    % this in theory should allow fmincon to use the interior-point algorithm
    % this line of code unintentionally made the simulation twice as fast
    coder.extrinsic('MPC_fmincon_u');
    coder.extrinsic('MPC_fmincon_x_u');
    coder.extrinsic("MPC_casadi_x_u");
    coder.extrinsic("MPC_fmincon_x_u_artificial_ref");
    
    % preinitialization
    deci_vars = zeros(size(prior_deci_vars, 1), 1);
    predicted_states_Nth_step = zeros(9, 1);
    desired_additional_thrust_and_body_rates = zeros(4, 1);
    iterations = 0;
    artifical_reference = zeros(4, 1);

    % timer
    MPC_start = tic;
   
    % if(solver == 1)
    %     [deci_vars,...
    %      predicted_states_Nth_step,...
    %      desired_additional_thrust_and_body_rates]  = MPC_quadprog(...
    %         prior_deci_vars,...
    %         x0,...
    %         v,...
    %         ssmodel,...
    %         weights,...
    %         constr_mat);
    
    if (solver == 2)
       [deci_vars,...
        predicted_states_Nth_step,...
        desired_additional_thrust_and_body_rates,...
        iterations]  = MPC_fmincon_x_u(...
            prior_deci_vars,...
            x0,...
            v,...
            ssmodel,...
            weights,....
            obs_params,...
            agent_params,...
            constr_mat,...
            safety_margin_universal, ...
            MPC_max_iters);

       % elseif (solver == 3)
       % 
       % [deci_vars,...
       %  predicted_states_Nth_step,...
       %  desired_additional_thrust_and_body_rates]  = MPC_fmincon_u(...
       %          prior_deci_vars,...
       %          weights,...
       %          x0,...
       %          v,...
       %          ssmodel,...
       %          lb,...
       %          ub,...
       %          H_MPC,...
       %          W_MPC);
    
    elseif (solver == 4)
       [deci_vars,...
        predicted_states_Nth_step,...
        desired_additional_thrust_and_body_rates]  = MPC_casadi_x_u(...
            prior_deci_vars,...
            x0,...
            v,...
            ssmodel,...
            weights,...
            obs_params,...
            agent_params,...
            constr_mat);
    elseif (solver == 5)
       [deci_vars,...
        predicted_states_Nth_step,...
        desired_additional_thrust_and_body_rates,...
        iterations]= MPC_fmincon_x_u_artificial_ref(...
            prior_deci_vars,...
            x0,...
            v,...
            ssmodel,...
            weights,....
            obs_params,...
            agent_params,...
            constr_mat,...
            safety_margin_universal, ...
            MPC_max_iters);
       artifical_reference(1:3, 1) = deci_vars(end-2:end, 1);
    end

    MPC_time = toc(MPC_start);

end

== matlab function Sim_quadrotor/Plant/Inner Controller (On-Board)/Inner Control Loop On-board/compute the per-propeller thrust desired ==
  data: cmd_per_motor_desired input; cmd_for_body_torques_desired input; cmd_to_apply output
function cmd_to_apply = distribute_power( cmd_per_motor_desired , cmd_for_body_torques_desired )
% ----------------------------------------------------------------------- %
% This function computes the uint16 command to apply to each motor as per
% the code that runs "on-board" on the Crazyflie's firmware
%
%
% INPUT ARGUMENTS:
%
% cmd_per_motor_desired [uint16]
% > This is a colulmn vector with length equal to the number of propellers
%   on the Crazyflie, i.e., 4, and each element represents the "baseline"
%   16-bit command that should be requested from the Crazyflie, as
%   requested by the outer loop controller.
%
% cmd_for_body_torques_desired [uint16]
% > This is the "actuation" uint16 command that comes directly from the
%   output of the Crazyflie's body rate PID controllers running in the
%   firmware. This value of command has already been adjust for the
%   dimensions of the Crazyflie, and the pattern for distributing the
%   command across the motor is provided in the exercise sheet.
%
%
% RETURN ARGUMENTS:
% % cmd_to_apply [uint16]
% > This is a colulmn vector with length equal to the number of propellers
%   on the Crazyflie, i.e., 4, and each element represents the 16-bit
%   command that will be requested from the motors
%
%
% DATA FORMAT ASSUMPTIONS:
% > the "cmd_per_motor_desired" vector is such when applied, the static
%   thrusts exert no torque about the body frame axes
%
% ----------------------------------------------------------------------- %

% cmd_per_motor_desired = double(cmd_per_motor_desired);
% cmd_for_body_torques_desired = double(cmd_for_body_torques_desired);

% Get the uint16 commands into a separate variable for each motor
cmd1 = cmd_per_motor_desired(1);
cmd2 = cmd_per_motor_desired(2);
cmd3 = cmd_per_motor_desired(3);
cmd4 = cmd_per_motor_desired(4);

if(cmd1 < 0 ||  cmd2 < 0 || cmd3 < 0 || cmd4 < 0)
    disp("negative cmd (addition thrust + mg) detected");
    cmd_per_motor_desired
end



% Get the desired body torques uint16 commands into a separate variable for
% the "uint16 command torque" desired about each of the body frame axes
r = cmd_for_body_torques_desired(1) / 2;
p = cmd_for_body_torques_desired(2) / 2;
y = cmd_for_body_torques_desired(3);


% These variable names have been used to partially match the code from the
% Crazyflie firmware:
% r  -  where "r" stands for roll, this is the "uint16 command torque" to
%       apply about the body-frame's x-axis, i.e., the roll-axis
% p  -  where "p" stands for pitch, this is the "uint16 command torque" to
%       apply about the body-frame's y-axis, i.e., the pitch-axis
% y  -  where "y" stands for yaw, this is the "uint16 command torque" to
%       apply about the body-frame's z-axis, i.e., the yaw-axis
%
% Note: the "/ 2" for the extraction of "r" and "p" above is simply added
% to minimic the code of the Crazyflie firmware. Presumably the Crazyflie's
% PID contollers for the body-frame roll and pitch axis are tuned with this
% factor of "/ 2" appropriately accounted for.


% Initialise the return variable "cmd_to_apply" to zeros
% > This can be required so that Simulink knows the expected size
cmd_to_apply = zeros(4,1);

% Compute the 16-bit command that should be applied from each motor as per
% the code from the Crazyflie firmware
% > For motor 1:
cmd_to_apply(1,1)  =  cmd1   - r   + p  +  y;
% > For motor 2:
cmd_to_apply(2,1)  =  cmd2   - r   - p  -  y;
% > For motor 3:
cmd_to_apply(3,1)  =  cmd3   + r   - p  +  y;
% > For motor 4:
cmd_to_apply(4,1)  =  cmd4   + r   + p  -  y;



if(cmd_to_apply(1,1) < 0 ||  cmd_to_apply(2,1) < 0 || cmd_to_apply(3,1) < 0 || cmd_to_apply(4,1) < 0)
    disp("inner controller negative cmd detected");
    cmd_to_apply
end

== matlab function Sim_quadrotor/Controller/MATLAB Function ==
  data: v input; x0 input; xi_N output; u_add output; K_lqr_outer_loop_discrete_time input
function [xi_N, u_add] = lqr(v, x0, K_lqr_outer_loop_discrete_time)
    xi_N = x0;
    x_bar_v = [v(1:3); zeros(5, 1); v(4)];
    u_add = -K_lqr_outer_loop_discrete_time * (x0 - x_bar_v);
    u_add = u_add(1:4);
end

== matlab function Sim_quadrotor/Plant/Quadrotor Vehicle Model (Plant)/plantModel ==
  data: full_state_dot output; thrusts input; full_state input; body_rates output; body_accel output; g parameter; layout_true parameter; inertia_true_inverse parameter; inertia_true parameter; mass_true parameter; A_continuous parameter; B_continuous parameter; time input
function [full_state_dot, body_rates, body_accel] = callPlantModel(...
    thrusts, ...
    full_state, ...
    g, ...
    layout_true, ...
    inertia_true_inverse, ...
    inertia_true, ...
    mass_true, ...
    A_continuous, ...
    B_continuous, ...
    time)

%% Note that the linear model is computed in a different branch inside the "plant" block. To switch between linear/nonlinear models, use the "inner_controller_inclusion" parameter.
    % disp("************Linear Model****************");
    % fprintf("time: %.5f", time);
    % [full_state_dot, body_rates, body_accel] = linearModel(thrusts, ...
    %     full_state, ...
    %     A_continuous, ...
    %     B_continuous, ...
    %     g, ...
    %     mass_true);


    % disp("------------Nonlinear Model------------")
    % fprintf("time: %.5f", time);
    [full_state_dot, body_rates, body_accel] = nonlinearModel(thrusts, ...
        full_state, ...
        g, ...
        mass_true, ...
        inertia_true, ...
        inertia_true_inverse, ...
        layout_true);

end

== matlab function Sim_quadrotor/Plant/Quadrotor Vehicle Model (Plant)1/MATLAB Function ==
  data: state input; state_dot output; control_input input; B_continuous_outer parameter; A_continuous_outer parameter
function state_dot = outerLoopEquations(state, control_input, B_continuous_outer, A_continuous_outer)

    state_dot = A_continuous_outer * state + B_continuous_outer * control_input;

end

== matlab function Sim_quadrotor/Plant/Sensors (On-Board and Off-Board)1/MATLAB Function ==
  data: mean input; noise_full_state_std_dev input; standard_normal_random input; random_sample output
function random_sample = sampling_from_multivariate_gaussian(mean, noise_full_state_std_dev, standard_normal_random)

random_sample = mean + noise_full_state_std_dev .* standard_normal_random;

end

== matlab function Sim_quadrotor/Plant/Sensors (On-Board and Off-Board)/MATLAB Function ==
  data: mean input; noise_full_state_std_dev input; standard_normal_random input; random_sample output
function random_sample = sampling_from_multivariate_gaussian(mean, noise_full_state_std_dev, standard_normal_random)

random_sample = mean + noise_full_state_std_dev .* standard_normal_random;

end

== matlab function Sim_quadrotor/Plant/Sensors (On-Board and Off-Board)/MATLAB Function1 ==
  data: mean input; covariance_decomposition input; standard_normal_random input; random_sample output
function random_sample = sampling_from_multivariate_gaussian(mean, covariance_decomposition, standard_normal_random)

random_sample = mean + covariance_decomposition * standard_normal_random;

== matlab function Sim_quadrotor/Plant/Sensors (On-Board and Off-Board)/MATLAB Function2 ==
  data: mean input; covariance_decomposition input; standard_normal_random input; random_sample output
function random_sample = sampling_from_multivariate_gaussian(mean, covariance_decomposition, standard_normal_random)

random_sample = mean + covariance_decomposition * standard_normal_random;

== matlab function Sim_quadrotor/Plant/compute_per_motor_thrust ==
  data: desired_thrusts_per_propeller output; additional_thrust_desired input; equilibrium_thrust parameter
function desired_thrusts_per_propeller = compute_per_motor_thrust(additional_thrust_desired,  equilibrium_thrust)

% This function compute the desired thrust per propeller

total_equilibrium_thrust = sum( equilibrium_thrust(:) );

desired_thrusts_per_propeller = equilibrium_thrust * ...
    ( (additional_thrust_desired + total_equilibrium_thrust) / ...
    total_equilibrium_thrust );
